simulink model "Auto_microgrid_forecasting_020322"  (R2020a)
settings: Solver=VariableStepAuto  StartTime=0.0  StopTime=10  MaxStep=1e-4  RelTol=1e-3
PreLoadFcn:
  | %run('FC_microgrid_param.m')
  | %load('gen_grid_init.mat')
InitFcn:
  | %load myisoModel_init;
  | run('FC_microgrid_param.m')
  | tic
  | run('CARTinitFcn.m')
  | %caseNo = 2;
  | 
  | %if (caseNo == 1)
  | %set_param(['Isolated_grid_paper_model_022521/SignalGen'], 'ActiveScenario', 'PStep222kW');
  | %else
  | %set_param(['Isolated_grid_paper_model_022521/SignalGen'], 'ActiveScenario', 'QStep222kVAr');
  | 
  | %end;
StopFcn:
  | toc
undefined symbols (not defined in the file or in its folder): breakpoints1, breakpoints2, cc_kp, cp_table_data, ctrl, D1, Delta, DiscIntNeverNeededParam, DT, FC_BESS, FC_PV_FirstSolar, find_system, Fnom, gcbh, libFC_BESS, libFC_PV, LowerLimit, magnitude, oversize, pll_ki, pll_kp, pq_ts, SOC_target, sps_rtmsupport, timer, Ts, ts, Ts_APC, Ts_Control, Ts_Power, UpperLimit
libraries: powerlib x151, simulink x100, powerlib_extras x100, powerlib_meascontrol x91, eePowerMeasurement x26, pi_ctrl x16, simulink_extras x12, sps_avr x7, spsDieselMotorModel x3, libFSArray x2, SignalEditorBlockLib x2, libLgBattery x1
(part 7 of 14)

== system Auto_microgrid_forecasting_020322/Stab1/AllStringInverters/Subsystem1 ==
  SmaINV : powerlib/Measurements/Three-Phase V-I Measurement  VoltageMeasurement=phase-to-ground  SetLabelV=off  LabelV=circuit_Usmainv  Vpu=off  VpuLL=off  CurrentMeasurement=yes  SetLabelI=off  LabelI=circuit_Ismainv  Ipu=off  Pbase=100e6  Vbase=500e3  OutputType=Complex  PhasorSimulation=off  PSBequivalent=0
  A : PMIOPort  Side=Left
  a : PMIOPort  Port=2  Side=Right
  B : PMIOPort  Port=3  Side=Left
  b : PMIOPort  Port=4  Side=Right
  C : PMIOPort  Port=5  Side=Left
  c : PMIOPort  Port=6  Side=Right
  tag scope: Iinv=scoped, Uinv=scoped
  wires:
  SmaINV/2 -> [Iinv]
  SmaINV/1 -> [Uinv]
  connections:
  A/RConn1 -- SmaINV/LConn1
  SmaINV/RConn3 -- c/RConn1
  SmaINV/RConn2 -- b/RConn1
  SmaINV/LConn2 -- B/RConn1
  C/RConn1 -- SmaINV/LConn3
  SmaINV/RConn1 -- a/RConn1

== system Auto_microgrid_forecasting_020322/Stab1/AllStringInverters/Subsystem2 ==
  GRI1 : powerlib/Measurements/Three-Phase V-I Measurement  VoltageMeasurement=phase-to-ground  SetLabelV=off  LabelV=Ugri  Vpu=off  VpuLL=off  CurrentMeasurement=yes  SetLabelI=off  LabelI=Igri  Ipu=off  Pbase=100e6  Vbase=500e3  OutputType=Complex  PhasorSimulation=off  PSBequivalent=0
  A : PMIOPort  Side=Left
  B : PMIOPort  Port=2  Side=Left
  a : PMIOPort  Port=3  Side=Right
  b : PMIOPort  Port=4  Side=Right
  C : PMIOPort  Port=5  Side=Left
  c : PMIOPort  Port=6  Side=Right
  tag scope: Igri=scoped, Ugri=scoped
  wires:
  GRI1/2 -> [Igri]
  GRI1/1 -> [Ugri]
  connections:
  GRI1/RConn1 -- a/RConn1
  GRI1/LConn1 -- A/RConn1
  GRI1/RConn2 -- b/RConn1
  GRI1/RConn3 -- c/RConn1
  GRI1/LConn2 -- B/RConn1
  GRI1/LConn3 -- C/RConn1

== system Auto_microgrid_forecasting_020322/Wind Turbine Type 4/APC (atomic)1/Baseline ==
  Action Port : ActionPort  ActionPortLabel=case [ 6 ]:
  Constant1 : Constant  Value=0
  Qcmd : Outport
  dP : Outport  Port=2
  dT : Outport  Port=3
  wires:
  Constant1/1 -> dP/1, dT/1, Qcmd/1

== system Auto_microgrid_forecasting_020322/Wind Turbine Type 4/APC (atomic)1/Inertial Response (to df) ==
  Freq (Hz) : Inport
  type1 : Inport  Port=2
  wg (pu) : Inport  Port=3
  f_setpoint : Inport  Port=4
  Action Port : ActionPort  ActionPortLabel=case [ 1 ]:
  Constant1 : Constant  Value=0
  Constant2 : Constant  Value=0
  Constant3 : Constant  Value=1e-3
  Display{3..4,6..7} (4 alike) : Display
  Divide1 : Product  Inputs=*/
  FBIC : Subsystem
  Gain : Gain  Gain=Fnom
  Lock2 : Subsystem
  Rate Limiter1 : RateLimiter  RisingSlewLimit=0.45  SampleTimeMode=inherited
  Relational Operator3 : RelationalOperator  OutDataTypeStr=boolean  RndMeth=Nearest
  Relational Operator4 : RelationalOperator  Operator=<=  OutDataTypeStr=boolean  RndMeth=Nearest
  Saturation : Saturate  UpperLimit=0.4  LowerLimit=0
  Saturation1 : Saturate  UpperLimit=1  LowerLimit=1e-5
  Scope : Scope  NumInputPorts=3
  Sum1 : Sum  Inputs=|-+
  Switch1 : Switch  Criteria=u2 > Threshold  Threshold=1
  TLIC : Subsystem  TreatAsAtomicUnit=on
  Type1 : Switch  Criteria=u2 > Threshold  Threshold=0.5
  When to start IR : DigitalClock  SampleTime=-1
  dead band1 : Constant  Value=0.2
  dT : Outport
  dP : Outport  Port=2
  Qcmd : Outport  Port=3
  wires:
  Constant1/1 -> dP/1, Qcmd/1
  Constant2/1 -> Switch1/3
  When to start IR/1 -> Switch1/2
  Lock2/1(O) -> Switch1/1
  Saturation/1 -> dT/1
  wg (pu)/1 -> [Wg], FBIC/1(wg (pu))
  Switch1/1 -> Display3/1, Scope/3, [In_Act]
  type1/1 -> Type1/2
  Sum1/1 -> Relational Operator3/1, Scope/2
  FBIC/1(Delta_P FBIC1) -> Type1/3
  Type1/1 -> [Delta_P], Display6/1
  Freq (Hz)/1 -> FBIC/2(Freq (Hz)1), [Freq]
  [In_Act] -> FBIC/3(Act1), TLIC/1(Act)
  TLIC/1(Delta_P TLIC) -> Type1/1
  [Delta_P] -> Relational Operator4/1
  f_setpoint/1 -> Gain/1
  dead band1/1 -> Relational Operator3/2
  Divide1/1 -> Rate Limiter1/1
  [Wg] -> Saturation1/1
  Saturation1/1 -> Divide1/2
  Constant3/1 -> Relational Operator4/2
  Relational Operator4/1 -> Display7/1, Lock2/2(R)
  [Freq] -> Sum1/1, Display4/1
  [Delta_P] -> Divide1/1, Scope/1
  Relational Operator3/1 -> Lock2/1(I)
  Rate Limiter1/1 -> Saturation/1
  Gain/1 -> Sum1/2

== system Auto_microgrid_forecasting_020322/Wind Turbine Type 4/APC (atomic)1/PFR ==
  Freq (Hz) : Inport
  f_setpoint : Inport  Port=2
  Action Port : ActionPort  ActionPortLabel=case [ 2 ]:
  Constant1 : Constant  Value=0
  Dead Zone : DeadZone  LowerValue=-db/60  UpperValue=db/60  SaturateOnIntegerOverflow=on
  Divide1 : Product  Inputs=*/
  Gain : Gain  Gain=Fnom
  P/f gain : Gain  Gain=1/k
  Saturation : Saturate  UpperLimit=0
  Sum : Sum  Inputs=|+-
  Sum1 : Sum  Inputs=|-+
  curtailment pu : Constant  Value=0.2
  dP : Outport
  dT : Outport  Port=2
  Qcmd : Outport  Port=3
  wires:
  Sum/1 -> Saturation/1
  Constant1/1 -> dT/1, Qcmd/1
  Saturation/1 -> dP/1
  P/f gain/1 -> Sum/1
  curtailment pu/1 -> Sum/2
  Dead Zone/1 -> P/f gain/1
  f_setpoint/1 -> Gain/1
  Freq (Hz)/1 -> Sum1/1
  Divide1/1 -> Dead Zone/1  "delta f pu"
  Sum1/1 -> Divide1/1
  Gain/1 -> Sum1/2, Divide1/2

== system Auto_microgrid_forecasting_020322/Wind Turbine Type 4/APC (atomic)1/PQ ==
  SFRcmd : Inport
  Qin : Inport  Port=2
  Action Port : ActionPort  ActionPortLabel=case [ 3 ]:
  Constant : Constant
  Constant1 : Constant  Value=0
  Sum : Sum  Inputs=|+-
  dP : Outport
  Qcmd : Outport  Port=2
  dT : Outport  Port=3
  wires:
  Constant1/1 -> dT/1
  Qin/1 -> Qcmd/1
  Constant/1 -> Sum/2
  Sum/1 -> dP/1
  SFRcmd/1 -> Sum/1

== system Auto_microgrid_forecasting_020322/Wind Turbine Type 4/APC (atomic)1/VR (handled by FRT) ==
  Action Port : ActionPort  ActionPortLabel=case [ 4 5 ]:
  Constant1 : Constant  Value=0
  Qcmd : Outport
  dP : Outport  Port=2
  dT : Outport  Port=3
  wires:
  Constant1/1 -> Qcmd/1, dT/1, dP/1

== system Auto_microgrid_forecasting_020322/Wind Turbine Type 4/Control/Excitation Control system ==
  Flux : Inport
  wr : Inport  Port=2
  Discrete PI Controller : Subsystem  DialogController=POWERSYS.PowerSysDialog  mask(Discrete PI Controller){Kp=Kp_field, Ki=Ki_field, Par_Limits=[1 0]*Vf_limit, Init=init(9), Ts=Ts}
      mask prompts: Kp "Proportional gain (Kp):"; Ki "Integral gain (Ki):"; Par_Limits "Output limits: [ Upper   Lower ]"; Init "Output initial value:"; Ts "Sample time:"
      mask help: This block implements a discrete PI controller.
      mask init:
      | UpperLimit=Par_Limits(1);
      | LowerLimit=Par_Limits(2);
      | power_initmask();
      mask Help: This block is part of a subset of blocks in the Extras library that does not have documentation associated with it, other than the block mask description.
      mask Display: disp('PI');
  Divide : Product  Inputs=*/
  Flux_ref : Constant
  "Flux_ref " : Constant
  Sum4 : Sum  Inputs=|+-  InputSameDT=on  SaturateOnIntegerOverflow=on  OutDataTypeStr=Inherit: Same as first input
  Switch : Switch  Threshold=1
  avoid division by 0 : Saturate  UpperLimit=inf  LowerLimit=1e-6
  Vf : Outport  VectorParamsAs1DForOutWhenUnconnected=off
  wires:
  Sum4/1 -> Discrete PI Controller/1(Error)
  Discrete PI Controller/1(Out) -> Vf/1  "Vf"
  Flux/1 -> Sum4/2  "Flux"
  wr/1 -> Switch/2, avoid division by 0/1
  Flux_ref/1 -> Switch/3
  "Flux_ref "/1 -> Divide/1
  avoid division by 0/1 -> Divide/2
  Divide/1 -> Switch/1
  Switch/1 -> Sum4/1

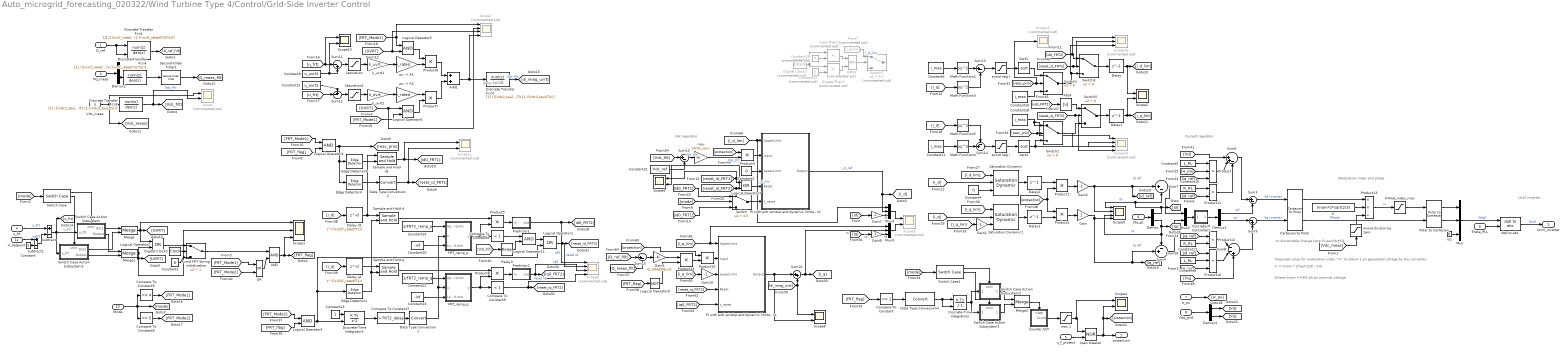
== system Auto_microgrid_forecasting_020322/Wind Turbine Type 4/Control/Grid-Side Inverter Control ==
  note: no discernable change here if use Vdc_filt
  note: di for FRT
  note: Required value for modulation index "m" to obtain 1 pu generated voltage by the converter:
  note: Modulation index and phase
  note: Where Vnom = RMS ph-ph nominal voltage
  note: Uctrl inverter
  note: Current regulator
  note: Iq ref
  note: m = Vnom * 2*sqrt(2/3) / Vdc
  note: Id ref
  note: Vdc regulator
  Q_ref : Inport
  PQ_meas : Inport  Port=2
  Vdc_meas : Inport  Port=3
  u_frt : Inport  Port=4
  u_f_protect : Inport  Port=5
  Idq_gc : Inport  Port=6
  w_pu : Inport  Port=7
  Vdq_grid : Inport  Port=8
  Theta_PLL : Inport  Port=9
  Mode : Inport  Port=10
  V_Setpoint : Inport  Port=11
  ->pu : Gain  Gain=1/Vdc_nom
  0-Mod_index_max : Saturate  UpperLimit=Mod_index_max  LowerLimit=0
  AND : Logic  IconShape=distinctive  AllPortsSameDT=off  OutDataTypeStr=boolean
  AND3 : Logic  Commented=on  IconShape=distinctive  AllPortsSameDT=off  OutDataTypeStr=boolean
  Abs4 : Abs
  Add1 : Sum
  Avoid FRT during initialization : Switch  Criteria=u2 > Threshold  Threshold=1
  Avoid division by zero : Saturate  UpperLimit=1e6  LowerLimit=1e-6
  Cartesian to Polar : simulink_extras/Transformations/Cartesian to Polar
  Compare To Constant : simulink/Logic and Bit Operations/Compare To Constant  relop===  const=1  OutDataTypeStr=boolean
  Compare To Constant5 : simulink/Logic and Bit Operations/Compare To Constant  relop===  const=4  OutDataTypeStr=boolean
  Compare To Constant6 : simulink/Logic and Bit Operations/Compare To Constant  relop===  const=5  OutDataTypeStr=boolean
  Compare To Constant7 : simulink/Logic and Bit Operations/Compare To Constant  relop=>  const=FRT2_delay  OutDataTypeStr=boolean
  Compare To Constant8 : simulink/Logic and Bit Operations/Compare To Constant  relop=<  const=1  OutDataTypeStr=boolean
  Compare To Constant9 : simulink/Logic and Bit Operations/Compare To Constant  relop=<  const=1  OutDataTypeStr=boolean
  Constant : Constant
  Constant10 : Constant  Value=R_RL
  Constant{6,11,16,18} (4 alike) : Constant  Value=i_max  SampleTime=Ts
  Constant12 : Constant  Value=u_ovrt1  SampleTime=Ts
  Constant13 : Constant
  Constant17 : Constant  Value=R_RL
  Constant19 : Constant  Value=1/FRT2_ramp_p  SampleTime=Ts
  Constant2 : Constant  Value=0  SampleTime=Ts
  Constant20 : Constant  Value=-inf  SampleTime=Ts
  Constant21 : Constant  Value=Vdc_ref  SampleTime=Ts
  Constant22 : Constant  Value=1/FRT2_ramp_q  SampleTime=Ts
  Constant23 : Constant  Value=-inf  SampleTime=Ts
  Constant27 : Constant  Commented=on  Value=2
  Constant28 : Constant  Commented=on  Value=7
  Constant3 : Constant  Value=0
  Constant4 : Constant  Value=0  SampleTime=Ts
  Constant5 : Constant  Value=L_RL
  Constant8 : Constant  Value=L_RL
  Constant9 : Constant  Value=u_uvrt1  SampleTime=Ts
  Counter AST : Subsystem
  Data Type Conversion1 : DataTypeConversion
  Data Type Conversion2 : DataTypeConversion
  Data Type Conversion4 : DataTypeConversion
  Delay{,1..3} (4 alike) : Delay  DelayLength=1  InitialCondition=0  SampleTime=Ts
  Delay d1 : Delay  DelayLength=fix(2/(f_rated*Ts))  InitialCondition=1  SampleTime=Ts
  Delay q1 : Delay  DelayLength=fix(2/(f_rated*Ts))  InitialCondition=1  SampleTime=Ts
  Demux{,2..4} (4 alike) : Demux  Outputs=2
      Demux settings: DisplayOption=none
      Demux3 settings: DisplayOption=none
      Demux4 settings: DisplayOption=none
  Digital Clock2 : DigitalClock  SampleTime=Ts
  Digital Clock3 : DigitalClock  Commented=on  SampleTime=-1
  Discrete PI Controller1 : Subsystem  DialogController=POWERSYS.PowerSysDialog  mask(Discrete PI Controller){Kp=Kp_grid_side_cur_reg, Ki=Ki_grid_side_cur_reg, Par_Limits=[1 -1]*Current_reg_output_limit, Init=0, Ts=Ts}
      mask prompts: Kp "Proportional gain (Kp):"; Ki "Integral gain (Ki):"; Par_Limits "Output limits: [ Upper   Lower ]"; Init "Output initial value:"; Ts "Sample time:"
      mask help: This block implements a discrete PI controller.
      mask init:
      | UpperLimit=Par_Limits(1);
      | LowerLimit=Par_Limits(2);
      | power_initmask();
      mask Help: This block is part of a subset of blocks in the Extras library that does not have documentation associated with it, other than the block mask description.
      mask Display: disp('PI');
  Discrete Transfer Fcn1 : DiscreteTransferFcn  Denominator=[(inv(f_rated)*2)/Ts (1-((inv(f_rated)*2)/Ts))]  InitialStatesSource=Input port  SampleTime=Ts
      settings: InputPortMap=u0,p5
  Discrete Transfer Fcn2 : DiscreteTransferFcn  Denominator=[(Vdc2_tau)/Ts (1-((Vdc2_tau)/Ts))]  InitialStates=Vdc2_filt_init  SampleTime=Ts
  Discrete Transfer Fcn3 : DiscreteTransferFcn  Denominator=[(Vdc2_tau)/Ts (1-((Vdc2_tau)/Ts))]  SampleTime=Ts
  Discrete Transfer Fcn4 : DiscreteTransferFcn  Denominator=[(inv(f_rated)*2)/Ts (1-((inv(f_rated)*2)/Ts))]  InitialStates=U_rated^2/(-inv(2*pi*f_rated*Cshunt_filter))  SampleTime=Ts
  Discrete-Time Integrator2 : DiscreteIntegrator  ExternalReset=falling  SampleTime=Ts  ICPrevOutput=DiscIntNeverNeededParam  ICPrevScaledInput=DiscIntNeverNeededParam
  Discrete-Time Integrator3 : DiscreteIntegrator  ExternalReset=level  SampleTime=Ts  LimitOutput=on  UpperSaturationLimit=1  LowerSaturationLimit=0  ICPrevOutput=DiscIntNeverNeededParam  ICPrevScaledInput=DiscIntNeverNeededParam
  Edge Detector1 : powerlib_meascontrol/Logic/Edge Detector  model=Rising  ic=0  Ts=Ts
      settings: SourceProductBaseCode=PS
  Edge Detector3 : powerlib_meascontrol/Logic/Edge Detector  model=Rising  ic=0  Ts=Ts
      settings: SourceProductBaseCode=PS
  Edge Detector4 : powerlib_meascontrol/Logic/Edge Detector  model=Falling  ic=0  Ts=Ts
      settings: SourceProductBaseCode=PS
  FRT_ramp_p : Subsystem
  FRT_ramp_q : Subsystem
  From7 : From  Commented=on  GotoTag=i_d_lim
  Gain : Gain
  Gain{1..2,7,10} (4 alike) : Gain  Gain=-1
  Gain5 : Gain  Gain=Q_rated/Nb_wt
  Gain9 : Gain
  GreaterThan2 : RelationalOperator  Commented=on  Operator=>  OutDataTypeStr=boolean  RndMeth=Simplest
  K : Constant  Value=Vnom*2*sqrt(2/3)
  Less Than2 : RelationalOperator  Commented=on  Operator=<  OutDataTypeStr=boolean  RndMeth=Simplest
  Logical Operator1 : Logic  Operator=OR  AllPortsSameDT=off  OutDataTypeStr=boolean
  Logical Operator{3..6,11} (5 alike) : Logic  AllPortsSameDT=off  OutDataTypeStr=boolean
  Logical Operator2 : Logic  Operator=OR  AllPortsSameDT=off  OutDataTypeStr=boolean
  Logical Operator7 : Logic  Operator=OR  AllPortsSameDT=off  OutDataTypeStr=boolean
  Logical Operator9 : Logic  Operator=NOT  AllPortsSameDT=off  OutDataTypeStr=boolean
  Math Function{2..5} (4 alike) : Math  Operator=magnitude^2  SignedPower=on  SaturateOnIntegerOverflow=on
  Merge : Merge
  Merge1 : Merge
  Merge2 : Merge
  Mux : Mux  Inputs=3
  Mux2 : Mux  Inputs=2
  Mux3 : Mux  Inputs=3
  Mux4 : Mux  Inputs=3
  OR : Logic  Operator=OR  IconShape=distinctive  AllPortsSameDT=off  OutDataTypeStr=boolean
  PI with anti-windup and dynamic limits - Id : Subsystem  mask(Discrete PI Controller with anti-windup and dynamic limiters){Kp=Kp_dc, Ki=Ki_dc, Init=Vdc_nom, Ts=Ts}
      mask prompts: Kp "Proportional gain (Kp):"; Ki "Integral gain (Ki):"; Init "State initial value:"; Ts "Sample time:"
      mask Display:
      | disp('PI-\nAST');
      | port_label('input',1,'Max');
      | port_label('input',2,'In');
      | port_label('input',3,'Min');
      | port_label('input',4,'Reset');
      | port_label('input',5,'x_reset');
      | port_label('output',1,'Out');
  PI with anti-windup and dynamic limits - Iq : Subsystem  mask(Discrete PI Controller with anti-windup and dynamic limiters){Kp=Q_Kp/1000, Ki=Q_Ki/1000, Init=0, Ts=Ts}
      mask prompts: Kp "Proportional gain (Kp):"; Ki "Integral gain (Ki):"; Init "State initial value:"; Ts "Sample time:"
      mask Display:
      | disp('PI-\nAST');
      | port_label('input',1,'Max');
      | port_label('input',2,'In');
      | port_label('input',3,'Min');
      | port_label('input',4,'Reset');
      | port_label('input',5,'x_reset');
      | port_label('output',1,'Out');
  Polar to Cartesian : simulink_extras/Transformations/Polar to Cartesian
      settings: SourceProductBaseCode=SL
  Predictor1 : Subsystem  mask{Init_value=0, Ts=Ts}
      mask prompts: Init_value "Initial value:"; Ts "Sample time (Ts):"
  Predictor2 : Subsystem  mask{Init_value=0, Ts=Ts}
      mask prompts: Init_value "Initial value:"; Ts "Sample time (Ts):"
  Product : Product  Inputs=3  InputSameDT=on  SaturateOnIntegerOverflow=on  OutDataTypeStr=Inherit: Same as first input
  Product{1..2,4..8,14..15} (9 alike) : Product
  Product10 : Product  Inputs=3  InputSameDT=on  SaturateOnIntegerOverflow=on  OutDataTypeStr=Inherit: Same as first input
  Product11 : Product  InputSameDT=on  SaturateOnIntegerOverflow=on  OutDataTypeStr=Inherit: Same as first input
  Product12 : Product  InputSameDT=on  SaturateOnIntegerOverflow=on  OutDataTypeStr=Inherit: Same as first input
  Product13 : Product  Inputs=**/  InputSameDT=on  SaturateOnIntegerOverflow=on  OutDataTypeStr=Inherit: Same as first input
  Relay3 : Relay  OnSwitchValue=1.02*Vdc_ref  OffSwitchValue=1.015*Vdc_ref  OutDataTypeStr=Inherit: Inherit via back propagation
  Sample and Hold d : powerlib_meascontrol/Additional Components/Sample and Hold  ic=0  Ts=Ts
      settings: SourceProductBaseCode=PS
  Sample and Hold d1 : powerlib_meascontrol/Additional Components/Sample and Hold  ic=0  Ts=Ts
      settings: SourceProductBaseCode=PS
  Sample and Hold q : powerlib_meascontrol/Additional Components/Sample and Hold  ic=0  Ts=Ts
      settings: SourceProductBaseCode=PS
  Saturation : Saturate  UpperLimit=0.08  LowerLimit=0
  Saturation Dynamic : simulink/Discontinuities/Saturation Dynamic  OutMin=[]  OutMax=[]  OutDataTypeStr=Inherit: Same as second input  OutDataType=fixdt(1, 16)  OutScaling=2^-10  DoSatur=off
  Saturation Dynamic1 : simulink/Discontinuities/Saturation Dynamic  OutMin=[]  OutMax=[]  OutDataTypeStr=Inherit: Same as second input  OutDataType=fixdt(1, 16)  OutScaling=2^-10  DoSatur=off
  Saturation1 : Saturate  UpperLimit=0  LowerLimit=-0.08
  Scope : Scope  Commented=on  NumInputPorts=2
  Scope1 : Scope  NumInputPorts=3
  Scope10 : Scope  Commented=on  NumInputPorts=4
  Scope11 : Scope  Commented=on  NumInputPorts=2
  Scope{2,4,6,9,13} (5 alike) : Scope  NumInputPorts=2
  Scope15 : Scope  Commented=on
  Scope16 : Scope  Commented=on  NumInputPorts=3
  Scope3 : Scope  Commented=on  NumInputPorts=2
  Scope5 : Scope  NumInputPorts=4
  Scope7 : Scope  Commented=on  NumInputPorts=4
  Scope8 : Scope  Commented=on  NumInputPorts=4
  Second-Order Filter1 : powerlib_meascontrol/Filters/Second-Order Filter  FilterType=Lowpass  Fo=Freq_filter  Zeta=Zeta_filter  Ts=Ts  Initialize=off  Vac_Init="[0,  0,  60]"  Vdc_Init=0  PlotResponse=off  FreqRange=[0, 500, 1]
      settings: SourceProductBaseCode=MT,PS
  Sqrt1 : Sqrt  SaturateOnIntegerOverflow=on
  Sqrt2 : Sqrt  SaturateOnIntegerOverflow=on
  Subtract : Sum  Inputs=+-
  Subtract1 : Sum  Inputs=+-
  Sum10 : Sum  Inputs=|+-
  Sum11 : Sum  Inputs=|-+
  Sum12 : Sum  Inputs=+-|
  Sum13 : Sum  Inputs=|+-
  Sum14 : Sum  Inputs=-+|
  Sum15 : Sum  Inputs=|+-
  Sum16 : Sum  Inputs=|++
  Sum3 : Sum  Inputs=|+-  InputSameDT=on  SaturateOnIntegerOverflow=on  OutDataTypeStr=Inherit: Same as first input
  Sum4 : Sum  Inputs=-+|  InputSameDT=on  SaturateOnIntegerOverflow=on  OutDataTypeStr=Inherit: Same as first input
  Sum6 : Sum  Inputs=||++-  InputSameDT=on  SaturateOnIntegerOverflow=on  OutDataTypeStr=Inherit: Same as first input
  Sum7 : Sum  Inputs=|+-  InputSameDT=on  SaturateOnIntegerOverflow=on  OutDataTypeStr=Inherit: Same as first input
  Sum8 : Sum  Inputs=|--+  InputSameDT=on  SaturateOnIntegerOverflow=on  OutDataTypeStr=Inherit: Same as first input
  Sum9 : Sum  Inputs=|-+  InputSameDT=on  SaturateOnIntegerOverflow=on  OutDataTypeStr=Inherit: Same as first input
  Switch : Switch  Criteria=u2 > Threshold  Threshold=4.5
  Switch Case : SwitchCase  CaseConditions={4, 5}
  Switch Case Action Subsystem : Subsystem  TreatAsAtomicUnit=on
  Switch Case Action Subsystem1 : Subsystem  TreatAsAtomicUnit=on
  Switch Case Action Subsystem2 : Subsystem  TreatAsAtomicUnit=on
  Switch Case Action Subsystem3 : Subsystem  TreatAsAtomicUnit=on
  Switch Case1 : SwitchCase  CaseConditions={4, 5}
  Switch{1..3,5} (4 alike) : Switch  Criteria=u2 > Threshold
  Switch7 : Switch  Commented=on  Criteria=u2 > Threshold  Threshold=0.5
  V0 : Constant  Value=0
  avoid neg i : Saturate  UpperLimit=i_max^2  LowerLimit=0
  avoid neg r : Saturate  UpperLimit=i_max^2  LowerLimit=0
  dq0 to abc : powerlib_meascontrol/Transformations/dq0 to abc  Alignment=90 degrees behind phase A axis
      settings: SourceProductBaseCode=MT,PS
  k_uvrt1 : Gain  Gain=k_uvrt
  k_uvrt2 : Gain  Gain=k_ovrt
  max 1 : Saturate  UpperLimit=1  LowerLimit=0
  open breaker : Logic  Operator=NOR  AllPortsSameDT=off  OutDataTypeStr=boolean
  "pu -> A1" : Gain  Gain=i_rated
  "pu -> A2" : Gain  Gain=i_rated
  protection : Outport
  Uctrl_inverter : Outport  Port=2  VectorParamsAs1DForOutWhenUnconnected=off
  wires:
  Logical Operator5/1 -> Product6/1
  [UVRT] -> Scope7/3, Logical Operator5/2
  [FRT_Mode1] -> Scope7/1, Logical Operator5/1
  Q_ref/1 -> Discrete Transfer Fcn1/1, Discrete Transfer Fcn1/2
  Discrete Transfer Fcn1/1 -> [Q_ref_filt]
  Product7/1 -> Add1/2
  "pu -> A2"/1 -> Product7/1
  Logical Operator6/1 -> Product7/2
  [FRT_Mode1] -> Logical Operator6/2
  [OVRT] -> Scope7/2, Logical Operator6/1
  Sum12/1 -> Saturation1/1
  k_uvrt2/1 -> "pu -> A2"/1
  Compare To Constant6/1 -> [FRT_Mode2]
  Compare To Constant5/1 -> [FRT_Mode1]
  [u_frt] -> Sum12/2
  Constant12/1 -> Sum12/1
  Add1/1 -> Scope7/4, Discrete Transfer Fcn3/1
  Product6/1 -> Add1/1
  "pu -> A1"/1 -> Product6/2
  Sum11/1 -> Saturation/1
  k_uvrt1/1 -> "pu -> A1"/1
  [u_frt] -> Scope13/1, Sum11/1
  Constant9/1 -> Scope13/2, Sum11/2
  Vdc_meas/1 -> Discrete Transfer Fcn2/1, Scope/1, [Vdc_meas]
  Discrete Transfer Fcn2/1 -> Scope/2, [Vdc_filt]  "Vdc_filt"
  Subtract/1 -> [u_frt], Switch Case Action Subsystem1/1(u_frt), Switch Case Action Subsystem/1(u_frt)  "u_Frt"
  Avoid FRT during initialization/1 -> AND/1
  avoid neg r/1 -> Sqrt1/1
  avoid neg i/1 -> Sqrt2/1
  [i_q] -> Math Function3/1
  [reac_prio] -> Scope10/3, Switch2/2
  Sqrt2/1 -> Scope10/2, Switch2/3
  Constant18/1 -> Scope10/1, Switch2/1
  [reac_prio] -> Scope15/1, Switch1/2
  Constant16/1 -> Switch1/3
  Sqrt1/1 -> Switch1/1
  [i_d] -> Math Function5/1
  Sum14/1 -> avoid neg i/1
  Constant11/1 -> Math Function4/1
  Sum13/1 -> avoid neg r/1
  Math Function3/1 -> Sum13/2
  Math Function2/1 -> Sum13/1
  Constant6/1 -> Math Function2/1
  Math Function4/1 -> Sum14/2
  Math Function5/1 -> Sum14/1
  Switch1/1 -> Switch3/3, Scope16/3
  Switch3/1 -> Delay/1
  [id0_FRT2] -> Scope16/1, Switch3/1
  [reset_id_FRT2] -> Scope16/2, Switch3/2
  Switch2/1 -> Switch5/3
  [iq0_FRT2] -> Abs4/1
  [reset_iq_FRT2] -> Scope10/4, Switch5/2
  Switch5/1 -> Delay1/1
  Delay/1 -> Scope2/1, [i_d_lim]
  Delay1/1 -> Scope2/2, [i_q_lim]
  Constant2/1 -> PI with anti-windup and dynamic limits - Id/3(LowerLimit)
  [i_q_lim] -> Gain1/1
  [i_q_lim] -> Saturation Dynamic1/1
  Gain1/1 -> Saturation Dynamic1/3
  [i_d_lim] -> Saturation Dynamic/1
  Saturation Dynamic1/1 -> Delay3/1
  Saturation Dynamic/1 -> Delay2/1
  Constant4/1 -> Saturation Dynamic/3
  PQ_meas/1 -> Demux2/1
  [i_d_lim] -> Mux4/1, PI with anti-windup and dynamic limits - Id/1(UpperLimit)  "i_d_lim"
  Demux2/2 -> Discrete Transfer Fcn4/1
  Abs4/1 -> Switch5/1
  [FRT_flag] -> Compare To Constant/1
  Discrete-Time Integrator2/1 -> Switch Case Action Subsystem2/1(u_frt), Switch Case Action Subsystem3/1(u_frt)
  Data Type Conversion4/1 -> Discrete-Time Integrator2/2, Discrete-Time Integrator2/1
  Merge2/1 -> Counter AST/Trigger
  Counter AST/1(Count) -> max 1/1
  Compare To Constant/1 -> Data Type Conversion4/1
  max 1/1 -> Scope4/1, open breaker/1
  u_f_protect/1 -> open breaker/2
  open breaker/1 -> protection/1, Scope4/2, [protection]
  [FRT_Mode2] -> Logical Operator4/1
  [FRT_flag] -> Logical Operator4/2
  [i_d] -> Delay d1/1
  [i_q] -> Delay q1/1
  Delay d1/1 -> Sample and Hold d1/1, Sample and Hold d/1
  Delay q1/1 -> Sample and Hold q/1
  Edge Detector1/1 -> Sample and Hold d/2, Sample and Hold q/2
  Constant13/1 -> Discrete-Time Integrator3/1
  Discrete-Time Integrator3/1 -> Compare To Constant7/1
  Compare To Constant7/1 -> Data Type Conversion1/1
  Product5/1 -> Predictor1/1(in)
  Product8/1 -> Predictor2/1(in)
  Sample and Hold q/1 -> Product8/1
  Predictor2/1(out) -> Scope8/3, [iq0_FRT2]  "iq0"
  FRT_ramp_q/1(y) -> Compare To Constant9/1, Product8/2
  Compare To Constant9/1 -> Scope8/4, [reset_iq_FRT2]  "reset iq"
  FRT_ramp_p/1(y) -> Compare To Constant8/1, Product5/2
  [Vdc_filt] -> Relay3/1
  Compare To Constant8/1 -> Logical Operator11/1
  Logical Operator11/1 -> Logical Operator1/1
  Logical Operator4/1 -> Discrete-Time Integrator3/2, Logical Operator1/2, Edge Detector1/1
  Logical Operator1/1 -> Scope8/2, [reset_id_FRT2]  "reset id"
  Data Type Conversion1/1 -> FRT_ramp_q/2(u), FRT_ramp_p/2(u)
  Relay3/1 -> Logical Operator11/2
  Constant19/1 -> FRT_ramp_p/1(UpperLimit)
  Constant20/1 -> FRT_ramp_p/3(LowerLimit)
  Constant22/1 -> FRT_ramp_q/1(UpperLimit)
  Constant23/1 -> FRT_ramp_q/3(LowerLimit)
  Switch/1 -> PI with anti-windup and dynamic limits - Id/5(x_reset)
  [FRT_Mode1] -> Logical Operator3/1
  [FRT_flag] -> Logical Operator3/2
  Logical Operator3/1 -> Edge Detector4/1, Edge Detector3/1, [reac_prio]
  Edge Detector3/1 -> Sample and Hold d1/2
  Sample and Hold d1/1 -> [id0_FRT1], Scope11/1
  Edge Detector4/1 -> Data Type Conversion2/1
  Data Type Conversion2/1 -> Scope11/2, [reset_id_FRT1]
  [reset_id_FRT1] -> Logical Operator7/1, Scope9/1
  [reset_id_FRT2] -> Scope9/2, Logical Operator7/2
  Logical Operator7/1 -> PI with anti-windup and dynamic limits - Id/4(Reset)
  [mode] -> Switch/2
  [id0_FRT1] -> Switch/3
  [id0_FRT2] -> Switch/1
  Predictor1/1(out) -> Scope8/1, [id0_FRT2]  "id0"
  Delay2/1 -> Product1/1
  Delay3/1 -> Product2/2
  [protection] -> Product2/1, Product1/2
  Product2/1 -> Gain/1
  Product4/1 -> PI with anti-windup and dynamic limits - Id/2(Input)
  [protection] -> Product4/1
  [i_d] -> Saturation Dynamic/2
  [i_q] -> Saturation Dynamic1/2
  Sample and Hold d/1 -> Product5/1
  Logical Operator2/1 -> Avoid FRT during initialization/1
  Constant3/1 -> Avoid FRT during initialization/3
  Digital Clock2/1 -> Avoid FRT during initialization/2
  [Vdc_meas] -> Avoid division by zero/1
  Cartesian to Polar/1 -> Product13/1
  Product13/1 -> 0-Mod_index_max/1  "m"
  Demux4/1 -> [Vd]
  w_pu/1 -> [w_pu]
  [iq_ref] -> Product/3
  Sum7/1 -> Mux2/1
  [w_pu] -> Product/2
  Product11/1 -> Sum6/3
  Avoid division by zero/1 -> Product13/3
  Product12/1 -> Sum8/1
  Demux3/2 -> Sum9/1  "vq'"
  Constant10/1 -> Product11/1
  Discrete PI Controller1/1(Out) -> Demux3/1
  Mux2/1 -> Discrete PI Controller1/1(Error)
  Product/1 -> Sum6/2
  Product1/1 -> Gain2/1
  Vdq_grid/1 -> Demux4/1
  Gain/1 -> Sum4/2, [iq_ref], Scope5/4
  Demux3/1 -> Sum3/2  "vd'"
  Constant8/1 -> Product10/2
  Product10/1 -> Sum8/2
  [Vd] -> Sum6/1
  Constant17/1 -> Product12/2
  [w_pu] -> Product10/3
  Sum8/1 -> Sum9/2
  Demux/1 -> Sum7/2, Scope5/1, [id]  "id"
  [id_ref] -> Product10/1
  dq0 to abc/1 -> Uctrl_inverter/1  "Uctrl"
  Polar to Cartesian/2 -> Mux/2
  Sum6/1 -> Sum3/1
  K/1 -> Product13/2
  Mux/1 -> dq0 to abc/1  "Vdq0"
  [Vq] -> Sum8/3
  Sum3/1 -> Cartesian to Polar/1  "Vd inverter"
  [iq_ref] -> Product12/1
  Cartesian to Polar/2 -> Polar to Cartesian/2  "Phase"
  0-Mod_index_max/1 -> Polar to Cartesian/1
  Sum9/1 -> Cartesian to Polar/2  "Vq inverter"
  [id_ref] -> Product11/2
  Constant5/1 -> Product/1
  Polar to Cartesian/1 -> Mux/1
  Sum4/1 -> Mux2/2
  Demux4/2 -> [Vq]
  V0/1 -> Mux/3
  Theta_PLL/1 -> dq0 to abc/2
  Idq_gc/1 -> Demux/1
  PI with anti-windup and dynamic limits - Id/1(Output) -> [i_d], Mux4/2  "i_d_ref"
  Gain2/1 -> Scope5/2, Sum7/1, [id_ref]
  ->pu/1 -> Product4/2  "Vdc_filt"
  Constant21/1 -> Sum10/2
  [Vdc_filt] -> Sum10/1
  Mux4/1 -> Scope3/1
  Mux3/1 -> Scope3/2
  Demux/2 -> Scope5/3, Sum4/1, [iq]  "iq"
  [id] -> Gain7/1
  Gain9/1 -> Mux3/3  "iq"
  Gain7/1 -> Mux4/3  "id"
  [iq] -> Gain9/1  "iq"
  [iq0_FRT2] -> PI with anti-windup and dynamic limits - Iq/5(x_reset)
  [FRT_flag] -> Logical Operator9/1
  [i_q_lim] -> Mux3/1, PI with anti-windup and dynamic limits - Iq/1(UpperLimit)
  PI with anti-windup and dynamic limits - Iq/1(Output) -> Scope6/2, Sum16/1
  Product14/1 -> Product15/2
  [Q_ref_filt] -> Sum15/1
  [reset_iq_FRT2] -> PI with anti-windup and dynamic limits - Iq/4(Reset)
  Logical Operator9/1 -> Product14/2
  Sum15/1 -> Gain5/1
  Sum16/1 -> Mux3/2, [i_q]  "iq"
  [Q_meas_filt] -> Sum15/2
  [i_q_lim] -> Gain10/1
  [di_imag_uvrt] -> Scope6/1, Sum16/2
  Product15/1 -> PI with anti-windup and dynamic limits - Iq/2(Input)
  [protection] -> Product15/1
  Gain10/1 -> PI with anti-windup and dynamic limits - Iq/3(LowerLimit)
  Saturation/1 -> k_uvrt1/1
  Saturation1/1 -> k_uvrt2/1
  Discrete Transfer Fcn3/1 -> [di_imag_uvrt]  "Vdc_filt"
  Sum10/1 -> ->pu/1  "Vdc_filt"
  Gain5/1 -> Product14/1
  Discrete Transfer Fcn4/1 -> Second-Order Filter1/1
  Second-Order Filter1/1 -> [Q_meas_filt]
  AND/1 -> Scope1/3, [FRT_flag]
  Digital Clock3/1 -> Less Than2/1, GreaterThan2/1
  Constant28/1 -> Less Than2/2
  Constant27/1 -> GreaterThan2/2
  From7/1 -> Switch7/1  "i_d_lim"
  AND3/1 -> Switch7/2
  GreaterThan2/1 -> AND3/2
  Less Than2/1 -> AND3/1
  [mode] -> Switch Case/1
  Switch Case/1 -> Switch Case Action Subsystem/Action
  Switch Case/2 -> Switch Case Action Subsystem1/Action
  Merge/1 -> Scope1/1, Logical Operator2/1, [OVRT]
  Switch Case Action Subsystem/1(Out1) -> Merge/1
  Switch Case Action Subsystem1/1(Out1) -> Merge/2
  Switch Case Action Subsystem/2(Output) -> Merge1/1
  Switch Case Action Subsystem1/2(Output) -> Merge1/2
  Merge1/1 -> Scope1/2, [UVRT], Logical Operator2/2
  Switch Case1/2 -> Switch Case Action Subsystem3/Action
  Switch Case1/1 -> Switch Case Action Subsystem2/Action
  [mode] -> Switch Case1/1
  Switch Case Action Subsystem2/1(Out1) -> Merge2/1
  Switch Case Action Subsystem3/1(Out1) -> Merge2/2
  u_frt/1 -> Subtract/1  "u_Frt"
  V_Setpoint/1 -> Subtract1/1
  Subtract1/1 -> Subtract/2  "u_Frt"
  Constant/1 -> Subtract1/2
  OR/1 -> AND/2
  Mode/1 -> [mode], Compare To Constant6/1, Compare To Constant5/1
  [FRT_Mode1] -> OR/1
  [FRT_Mode2] -> OR/2

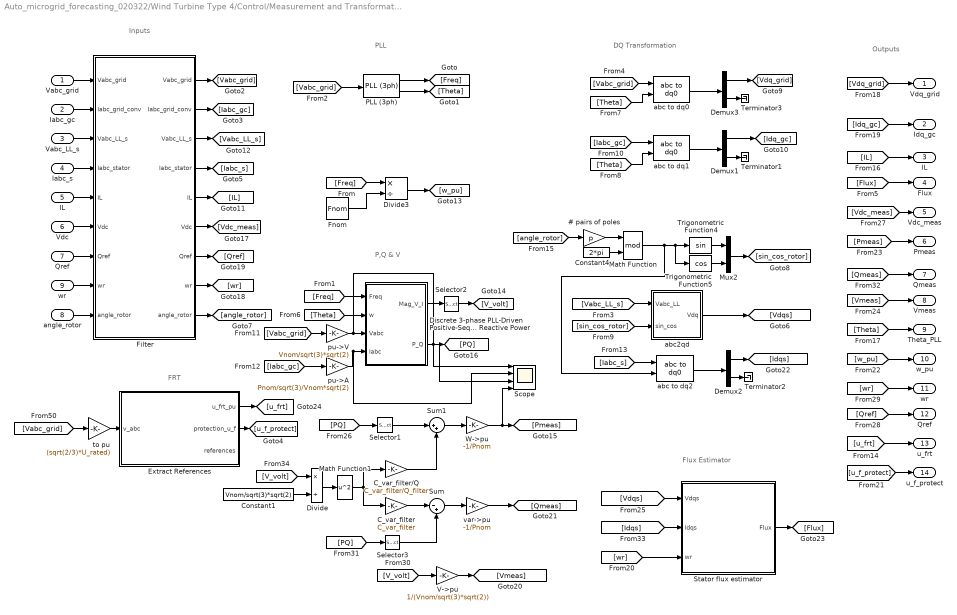
== system Auto_microgrid_forecasting_020322/Wind Turbine Type 4/Control/Measurement and Transformation ==
  note: Flux Estimator
  note: Outputs
  note: PLL
  note: DQ Transformation
  note: P,Q & V
  note: Inputs
  note: FRT
  Vabc_grid : Inport
  Iabc_gc : Inport  Port=2
  Vabc_LL_s : Inport  Port=3
  Iabc_s : Inport  Port=4
  IL : Inport  Port=5
  Vdc : Inport  Port=6
  Qref : Inport  Port=7
  angle_rotor : Inport  Port=8
  wr : Inport  Port=9
  # pairs of poles : Gain  Gain=p  SaturateOnIntegerOverflow=on  OutDataTypeStr=Inherit: Same as input  ParamDataTypeStr=Inherit: Same as input
  C_var_filter : Gain  Gain=C_var_filter  SaturateOnIntegerOverflow=on  OutDataTypeStr=Inherit: Same as input  ParamDataTypeStr=Inherit: Same as input
  C_var_filter/Q : Gain  Gain=C_var_filter/Q_filter  SaturateOnIntegerOverflow=on  OutDataTypeStr=Inherit: Same as input  ParamDataTypeStr=Inherit: Same as input
  Constant1 : Constant  Value=Vnom/sqrt(3)*sqrt(2)
  Constant4 : Constant  Value=2*pi
  Demux1 : Demux  Outputs=[2 1]
      settings: DisplayOption=none
  Demux2 : Demux  Outputs=[2 1]
      settings: DisplayOption=none
  Demux3 : Demux  Outputs=[2 1]
      settings: DisplayOption=none
  Discrete 3-phase PLL-Driven Positive-Sequence Active & Reactive Power : Subsystem  mask(Discrete 3-phase PLL-Driven Positive-Sequence Active & Reactive Power){Finit=Fnom, Fmin=Fnom*45/60, Par_Vinit=[Vnom/sqrt(3)*sqrt(2) 30], Par_Iinit=[Pnom/sqrt(3)/Vnom*sqrt(2) -10], Ts=Ts}
      mask prompts: Finit "Initial frequency (Hz):"; Fmin "Minimum frequency (Hz):"; Par_Vinit "Voltage initial input: [ Mag  Phase(Degrees) ]"; Par_Iinit "Current initial input: [ Mag  Phase(Degrees) ]"; Ts "Sample time:"
      mask help:
      | This discrete block measures the 3-phase active power P and reactive power Q  associated with a periodic set of 3-phase voltages and currents which may contain harmonics. P and Q are calculated by evaluating the fundamental values (positive-sequence) of the input voltages and currents with a running window over one cycle of the specified frequency (port Freq).
      |  Input port "Sin_Cos" (a two-dimension signal) provides the reference frame required for the computation.
      |
      | input 1: must give the frequency of the fundamental (Hz)
      | Input 2: must contain a  [sin(wt)  cos(wt)] two dimension signal , where w is the rotation speed (rad/s) of the reference frame used for the computation..
      | input 3: Vectorized 3-phase  instantaneous voltage (Vabc)
      | input 4: Vectorized 3-phase instantaneous current (Iabc)
      |
      | Output 1: Vector [Mag_V Mag_I] of the fundamental values (Magnitude) of the voltage & current (peak values of the positive-sequence)
      | Output 2: 3-phase PQ measurement vector [P(W) Q (var)] evaluated at the specified frequency. Current flowing into an RL circuit will produce  positive active and reactive powers.
      |
      | For the first cycle of simulation, the outputs are held constant using the values specified by the parameters "Initial input".
      | he value of the parameter "Minimum frequency" is used to determine the buffer size of the "Variable Transport Delay" block found inside this subsystem.
      mask init:
      | power_initmask();
      settings: OpenFcn=power_openblockproxy();
  Divide : Product  Inputs=*/
  Divide3 : Product  Inputs=*/
  Extract References : Subsystem
  Filter : Subsystem  mask{Freq=Freq_filter, Zeta=Zeta_filter, Ts=Ts}
      mask prompts: Freq "Cut-off frequency (Hz):"; Zeta "Damping factor Zeta:"; Ts "Sample time"
  Fnom : Constant  Value=Fnom
  Math Function : Math  Operator=mod  SignedPower=on  SaturateOnIntegerOverflow=on
  Math Function1 : Math  Operator=square  SignedPower=on  SaturateOnIntegerOverflow=on
  Mux2 : Mux  Inputs=2
  PLL (3ph) : powerlib_meascontrol/PLL/PLL (3ph)  Fmin=0.75*Fnom  Par_Init=[-45 Fnom]  ParK=[60 1400 1]  TcD=1e-4  MaxRateChangeFreq=12  FilterCutOffFreq=25  Ts=Ts  AGC=on
      settings: SourceProductBaseCode=MT,PS
  Scope : Scope  NumInputPorts=4
  Selector1 : Selector  InputPortWidth=2  IndexOptions=Index vector (dialog)  Indices=1  OutputSizes=1
  Selector2 : Selector  InputPortWidth=2  IndexOptions=Index vector (dialog)  Indices=1  OutputSizes=1
  Selector3 : Selector  InputPortWidth=2  IndexOptions=Index vector (dialog)  Indices=2  OutputSizes=1
  Stator flux estimator : Subsystem
  Sum : Sum  Inputs=|-+
  Sum1 : Sum  Inputs=|++
  Terminator1 : Terminator
  Terminator2 : Terminator
  Terminator3 : Terminator
  Trigonometric Function4 : Trigonometry
  Trigonometric Function5 : Trigonometry  Operator=cos
  V->pu : Gain  Gain=1/(Vnom/sqrt(3)*sqrt(2))  SaturateOnIntegerOverflow=on  OutDataTypeStr=Inherit: Same as input  ParamDataTypeStr=Inherit: Same as input
  W->pu : Gain  Gain=-1/Pnom  SaturateOnIntegerOverflow=on  OutDataTypeStr=Inherit: Same as input  ParamDataTypeStr=Inherit: Same as input
  abc to dq0 : powerlib_meascontrol/Transformations/abc to dq0  Alignment=90 degrees behind phase A axis
      settings: SourceProductBaseCode=MT,PS
  abc to dq1 : powerlib_meascontrol/Transformations/abc to dq0  Alignment=90 degrees behind phase A axis
      settings: SourceProductBaseCode=MT,PS
  abc to dq2 : powerlib_meascontrol/Transformations/abc to dq0  Alignment=90 degrees behind phase A axis
      settings: SourceProductBaseCode=MT,PS
  abc2qd : Subsystem
  pu->A : Gain  Gain=Pnom/sqrt(3)/Vnom*sqrt(2)  SaturateOnIntegerOverflow=on  OutDataTypeStr=Inherit: Same as input  ParamDataTypeStr=Inherit: Same as input
  pu->V : Gain  Gain=Vnom/sqrt(3)*sqrt(2)  SaturateOnIntegerOverflow=on  OutDataTypeStr=Inherit: Same as input  ParamDataTypeStr=Inherit: Same as input
  to pu : Gain  Gain=(sqrt(2/3)*U_rated)
  "var->pu " : Gain  Gain=-1/Pnom  SaturateOnIntegerOverflow=on  OutDataTypeStr=Inherit: Same as input  ParamDataTypeStr=Inherit: Same as input
  Vdq_grid : Outport  VectorParamsAs1DForOutWhenUnconnected=off
  Idq_gc : Outport  Port=2  VectorParamsAs1DForOutWhenUnconnected=off
  "IL " : Outport  Port=3  VectorParamsAs1DForOutWhenUnconnected=off
  Flux : Outport  Port=4  VectorParamsAs1DForOutWhenUnconnected=off
  Vdc_meas : Outport  Port=5  VectorParamsAs1DForOutWhenUnconnected=off
  Pmeas : Outport  Port=6  VectorParamsAs1DForOutWhenUnconnected=off
  Qmeas : Outport  Port=7  VectorParamsAs1DForOutWhenUnconnected=off
  Vmeas : Outport  Port=8  VectorParamsAs1DForOutWhenUnconnected=off
  Theta_PLL : Outport  Port=9  VectorParamsAs1DForOutWhenUnconnected=off
  w_pu : Outport  Port=10  VectorParamsAs1DForOutWhenUnconnected=off
  "wr " : Outport  Port=11  VectorParamsAs1DForOutWhenUnconnected=off
  "Qref " : Outport  Port=12  VectorParamsAs1DForOutWhenUnconnected=off
  u_frt : Outport  Port=13
  u_f_protect : Outport  Port=14
  wires:
  Filter/9("angle_rotor ") -> [angle_rotor]
  angle_rotor/1 -> Filter/9(angle_rotor)
  Stator flux estimator/1(Flux) -> [Flux]
  # pairs of poles/1 -> Math Function/1
  Constant4/1 -> Math Function/2
  abc2qd/1(Vdq) -> [Vdqs]
  Trigonometric Function5/1 -> Mux2/2
  Trigonometric Function4/1 -> Mux2/1
  [angle_rotor] -> # pairs of poles/1
  [Vabc_LL_s] -> abc2qd/1(Vabc_LL)
  [sin_cos_rotor] -> abc2qd/2(sin_cos)
  Mux2/1 -> [sin_cos_rotor]
  Demux2/1 -> [Idqs]
  Demux2/2 -> Terminator2/1
  abc to dq2/1 -> Demux2/1
  [Iabc_s] -> abc to dq2/1
  [Vdqs] -> Stator flux estimator/1(Vdqs)
  [Idqs] -> Stator flux estimator/2(Idqs)
  [wr] -> Stator flux estimator/3(wr)
  [Qmeas] -> Qmeas/1
  "var->pu "/1 -> [Qmeas]
  [PQ] -> Selector3/1
  V->pu/1 -> [Vmeas]
  [V_volt] -> V->pu/1
  Selector2/1 -> [V_volt]
  Discrete 3-phase PLL-Driven Positive-Sequence Active & Reactive Power/1(Mag_V_I) -> Selector2/1
  Demux1/2 -> Terminator1/1
  Demux3/1 -> [Vdq_grid]
  Demux3/2 -> Terminator3/1
  abc to dq1/1 -> Demux1/1
  abc to dq0/1 -> Demux3/1
  PLL (3ph)/1 -> [Freq]
  Fnom/1 -> Divide3/2
  Divide3/1 -> [w_pu]
  pu->V/1 -> Scope/1, Discrete 3-phase PLL-Driven Positive-Sequence Active & Reactive Power/3(Vabc)
  W->pu/1 -> Scope/4, [Pmeas]
  [Freq] -> Divide3/1
  [Freq] -> Discrete 3-phase PLL-Driven Positive-Sequence Active & Reactive Power/1(Freq)
  PLL (3ph)/2 -> [Theta]
  [Vabc_grid] -> abc to dq0/1
  [Theta] -> Discrete 3-phase PLL-Driven Positive-Sequence Active & Reactive Power/2(w)
  [Theta] -> abc to dq0/2
  [Theta] -> abc to dq1/2
  [Vabc_grid] -> PLL (3ph)/1
  [Iabc_gc] -> abc to dq1/1
  [Theta] -> Theta_PLL/1
  Demux1/1 -> [Idq_gc]
  [Vdq_grid] -> Vdq_grid/1
  [Idq_gc] -> Idq_gc/1
  [w_pu] -> w_pu/1
  [Pmeas] -> Pmeas/1
  [Vmeas] -> Vmeas/1
  pu->A/1 -> Discrete 3-phase PLL-Driven Positive-Sequence Active & Reactive Power/4(Iabc), Scope/2
  [PQ] -> Selector1/1
  [Vdc_meas] -> Vdc_meas/1
  [Qref] -> "Qref "/1
  [wr] -> "wr "/1
  [Flux] -> Flux/1
  [Vabc_grid] -> pu->V/1
  [Iabc_gc] -> pu->A/1
  Discrete 3-phase PLL-Driven Positive-Sequence Active & Reactive Power/2(P_Q) -> Scope/3, [PQ]
  Vabc_grid/1 -> Filter/1(Vabc_grid)
  Vdc/1 -> Filter/6(Vdc)
  Qref/1 -> Filter/7(Qref)
  wr/1 -> Filter/8(wr)
  Filter/1("Vabc_grid ") -> [Vabc_grid]
  Filter/2("Iabc_grid_conv ") -> [Iabc_gc]
  Filter/4("Iabc_stator ") -> [Iabc_s]
  Filter/6("Vdc ") -> [Vdc_meas]
  Filter/8("wr ") -> [wr]
  Filter/7("Qref ") -> [Qref]
  Iabc_gc/1 -> Filter/2(Iabc_grid_conv)
  Iabc_s/1 -> Filter/4(Iabc_stator)
  Vabc_LL_s/1 -> Filter/3(Vabc_LL_s)
  Filter/3("Vabc_LL_s ") -> [Vabc_LL_s]
  [V_volt] -> Divide/1
  Constant1/1 -> Divide/2
  Divide/1 -> Math Function1/1
  Selector3/1 -> Sum/2
  C_var_filter/1 -> Sum/1
  Sum/1 -> "var->pu "/1
  Math Function1/1 -> C_var_filter/Q/1, C_var_filter/1
  Selector1/1 -> Sum1/1
  C_var_filter/Q/1 -> Sum1/2
  Sum1/1 -> W->pu/1
  IL/1 -> Filter/5(IL)
  Filter/5("IL ") -> [IL]
  [IL] -> "IL "/1
  Math Function/1 -> abc to dq2/2, Trigonometric Function5/1, Trigonometric Function4/1
  Extract References/1(u_frt_pu) -> [u_frt]
  Extract References/2(protection_u_f) -> [u_f_protect]
  [Vabc_grid] -> to pu/1
  [u_frt] -> u_frt/1
  [u_f_protect] -> u_f_protect/1
  to pu/1 -> Extract References/1(v_abc)

== system Auto_microgrid_forecasting_020322/Wind Turbine Type 4/Control/Speed & Pitch Control3 ==
  note: Current Regulator
  note: Note :
      | This control system is based on the report:
      | Dynamic Modeling of GE 1.5 and 3.6 Wind Turbine-Generators;
      | Prepared by: Nicholas W. Miller, William W. Price, Juan J. Sanchez-Gasca;
      | October 27, 2003, Version 3.0
      | GE-Power Systems Energy Consulting
      | Copyright 2002 General Electric Company, U.S.A.
      |
      | Another reference is:
      |
      | DYNAMIC MODELING OF GE 1.5 AND 3.6 MW WIND TURBINE GENERATORS
      | FOR STABILITY SIMULATIONS
      | Nicholas W. Miller, Juan J. Sanchez-Gasca, William W. Price Robert W. Delmerico
      | GE Power Systems GE Research
      | Schenectady, NY Niskayuna, NY
      |
      | 0-7803-7989-6/03/$17.00 02003 IEEE
  note: Speed Regulator
  note: Pitch Compensation
  note: Pitch Control
  wr : Inport
  Pmeas : Inport  Port=2
  IL : Inport  Port=3
  Tgain : Inport  Port=4
  Pref : Inport  Port=5
  U5s1 : Inport  Port=6
  0-inf : Saturate  UpperLimit=inf  LowerLimit=0
  0-pitch_max : Saturate  UpperLimit=pitch_max  LowerLimit=0
  "0-pitch_max " : Saturate  UpperLimit=pitch_max  LowerLimit=0
  Constant1 : Constant
  Delay1 : Delay  DelayLength=1  InitialCondition=2
  Discrete PI Controller1 : Subsystem  DialogController=POWERSYS.PowerSysDialog  mask(Discrete PI Controller){Kp=Kp_compensation, Ki=Ki_compensation, Par_Limits=[pitch_max 0], Init=0, Ts=Ts}
      mask prompts: Kp "Proportional gain (Kp):"; Ki "Integral gain (Ki):"; Par_Limits "Output limits: [ Upper   Lower ]"; Init "Output initial value:"; Ts "Sample time:"
      mask help: This block implements a discrete PI controller.
      mask init:
      | UpperLimit=Par_Limits(1);
      | LowerLimit=Par_Limits(2);
      | power_initmask();
      mask Help: This block is part of a subset of blocks in the Extras library that does not have documentation associated with it, other than the block mask description.
      mask Display: disp('PI');
  Discrete PI Controller2 : Subsystem  DialogController=POWERSYS.PowerSysDialog  mask(Discrete PI Controller){Kp=Kp_boost_cur_reg*1, Ki=Ki_boost_cur_reg*0.005, Par_Limits=[1 0], Init=0.5, Ts=Ts}
      mask prompts: Kp "Proportional gain (Kp):"; Ki "Integral gain (Ki):"; Par_Limits "Output limits: [ Upper   Lower ]"; Init "Output initial value:"; Ts "Sample time:"
      mask help: This block implements a discrete PI controller.
      mask init:
      | UpperLimit=Par_Limits(1);
      | LowerLimit=Par_Limits(2);
      | power_initmask();
      mask Help: This block is part of a subset of blocks in the Extras library that does not have documentation associated with it, other than the block mask description.
      mask Display: disp('PI');
  First-Order Filter : powerlib_meascontrol/Filters/First-Order Filter  FilterType=Lowpass  Tc=Pitch_time_constant  Ts=Ts  Initialize=on  Vac_Init=[0.8 -25 60]*0  Vdc_Init=0  PlotResponse=off  FreqRange="[0,  200,  1]"
      settings: SourceProductBaseCode=MT,PS
  First-Order Filter1 : powerlib_meascontrol/Filters/First-Order Filter  FilterType=Lowpass  Tc=T_speed  Ts=Ts  Initialize=on  Vac_Init=[0, 0, 0]  Vdc_Init=1+init(1)/100  PlotResponse=off  FreqRange="[0,  200,  1]"
      settings: SourceProductBaseCode=MT,PS
  Gain2 : Gain  Gain=Kp_pitch  SaturateOnIntegerOverflow=on  OutDataTypeStr=Inherit: Same as input  ParamDataTypeStr=Inherit: Same as input
  Less Than : RelationalOperator  Operator=<=  OutDataTypeStr=boolean  RndMeth=Simplest
  MATLAB Function1 : MATLAB Function  TreatAsAtomicUnit=on
  Merge1 : Merge  Inputs=3
  Operational1 : Subsystem  TreatAsAtomicUnit=on
  PID Controller1 : simulink/Continuous/PID Controller  Controller=PI  Form=Parallel  TimeDomain=Discrete-time  UseExternalTs=off  SampleTime=-1  IntegratorMethod=Forward Euler  FilterMethod=Forward Euler  ControllerParametersSource=internal  P=Kp_speed  I=Ki_speed  D=0  UseFilter=on  N=100  TunerSelectOption=Transfer Function Based (PID Tuner App)  InitialConditionSource=internal  InitialConditionForIntegrator=0  InitialConditionForFilter=0  DifferentiatorICPrevScaledInput=0  ExternalReset=none  TrackingMode=off  Kt=1  LimitOutput=on  UpperSaturationLimit=1.  LowerSaturationLimit=0.8  LinearizeAsGain=on  AntiWindupMode=back-calculation  Kb=1e4  POutMin=[]  POutMax=[]  IOutMin=[]  IOutMax=[]  DOutMin=[]  DOutMax=[]  NOutMin=[]  NOutMax=[]  SumOutMin=[]  SumOutMax=[]  SaturationOutMin=[]  SaturationOutMax=[]  PParamMin=[]  PParamMax=[]  IParamMin=[]  IParamMax=[]  DParamMin=[]  DParamMax=[]  NParamMin=[]  NParamMax=[]  KbParamMin=[]  KbParamMax=[]  KtParamMin=[]  KtParamMax=[]  KbOutMin=[]  KbOutMax=[]  KtOutMin=[]  KtOutMax=[]  IntegratorOutMin=[]  IntegratorOutMax=[]  FilterOutMin=[]  FilterOutMax=[]  SumI1OutMin=[]  SumI1OutMax=[]  SumI2OutMin=[]  SumI2OutMax=[]  SumI3OutMin=[]  SumI3OutMax=[]  SumI4OutMin=[]  SumI4OutMax=[]  SumDOutMin=[]  SumDOutMax=[]  DifferentiatorOutMin=[]  DifferentiatorOutMax=[]  FilterDiffOutCoefMin=[]  FilterDiffOutCoefMax=[]  ReciprocalOutMin=[]  ReciprocalOutMax=[]  SumDenOutMin=[]  SumDenOutMax=[]  SumNumOutMin=[]  SumNumOutMax=[]  DivideOutMin=[]  DivideOutMax=[]  UdiffTsProdOutMin=[]  UdiffTsProdOutMax=[]  NTsProdOutMin=[]  NTsProdOutMax=[]  UintegralTsProdOutMin=[]  UintegralTsProdOutMax=[]  UngainTsProdOutMin=[]  UngainTsProdOutMax=[]  IntegratorContinuousStateAttributes=''  IntegratorStateMustResolveToSignalObject=off  IntegratorRTWStateStorageClass=Auto  FilterContinuousStateAttributes=''  FilterStateMustResolveToSignalObject=off  FilterRTWStateStorageClass=Auto  ParallelPVariant=InternalParameters  IdealPVariant=Disabled  IVariant=InternalParameters  DVariant=Disabled  IntegratorVariant=Discrete  SatVariant=Enabled  AWVariant=BackCalculation  PCopyVariant=Disabled  TRVariant=Disabled  FdbkBlocksVariant=Forward  IdealPFdbkVariant=Disabled  SatFdbkVariant=Disabled  DerivativeFilterVariant=Disabled  NVariant=Disabled  NCopyVariant=Disabled_SignalSpec  FilterICVariant=Disabled  IntegratorICVariant=InternalICs  ExternalResetVariant=Disabled  TRSumVariant=Passthrough  SumFdbkVariant=Disabled  SumVariant=Sum_PI  TsampFilterVariant=InternalTs  TsampNgainVariant=Passthrough  TsampIntegralVariant=Passthrough
  Rate Limiter   1 : RateLimiter  RisingSlewLimit=pitch_rate  FallingSlewLimit=-pitch_rate
  Scope1 : Scope  NumInputPorts=6
  Scope4 : Scope  NumInputPorts=4
  Shutdown1 : Subsystem  TreatAsAtomicUnit=on
  Startup1 : Subsystem  TreatAsAtomicUnit=on
  Sum : Sum  Inputs=-+  SaturateOnIntegerOverflow=on
  Sum1 : Sum  Inputs=|+-
  Sum2 : Sum  Inputs=|+-  SaturateOnIntegerOverflow=on
  Sum3 : Sum  Inputs=|++
  Sum4 : Sum  Inputs=|+-
  Switch : Switch  Threshold=0.75
  Switch Case1 : SwitchCase  CaseConditions={1, 2, 3}
  Switch1 : Switch  Criteria=u2 > Threshold  Threshold=0.5
  Tracking Curve : Fcn  Expr=-0.5551*u(1)^2+1.183*u(1)+0.425
  pu_elec->pu_mec : Gain  Gain=Pnom/Pmec
  wref : Constant
  Duty_Cycle : Outport  VectorParamsAs1DForOutWhenUnconnected=off
  Pitch (deg) : Outport  Port=2  VectorParamsAs1DForOutWhenUnconnected=off
  wires:
  First-Order Filter/1 -> Operational1/1(In1)  "Pitch"
  MATLAB Function1/1(state) -> Delay1/1, Scope4/1, Switch Case1/1  "state"
  Delay1/1 -> MATLAB Function1/3("state ")
  Switch Case1/1 -> Startup1/Action
  Startup1/1(Out1) -> Merge1/1
  [wr] -> MATLAB Function1/2(wr), Scope4/3  "wr"
  U5s1/1 -> MATLAB Function1/1(U5s), Scope4/2  "U5s"
  Switch Case1/2 -> Operational1/Action
  Merge1/1 -> Pitch (deg)/1, Scope4/4  "pitch"
  Shutdown1/1(Out1) -> Merge1/3
  Switch Case1/3 -> Shutdown1/Action
  Operational1/1(Out1) -> Merge1/2
  PID Controller1/1 -> Switch1/1  "ILref"
  Less Than/1 -> Switch1/2
  Constant1/1 -> Less Than/2
  Tgain/1 -> Less Than/1, Switch1/3
  Switch1/1 -> Sum4/1, Scope1/4  "ILref"
  Discrete PI Controller2/1(Out) -> Duty_Cycle/1, Scope1/6  "Duty cycle"
  IL/1 -> Sum4/2, Scope1/5  "IL"
  Sum4/1 -> Discrete PI Controller2/1(Error)
  Tracking Curve/1 -> Switch/3
  First-Order Filter1/1 -> Sum/1, Sum1/2, Scope1/1  "wref"
  Sum2/1 -> Discrete PI Controller1/1(Error)
  Sum/1 -> Gain2/1
  "0-pitch_max "/1 -> First-Order Filter/1
  0-pitch_max/1 -> Sum3/1  "Pitch_contrl"
  Pmeas/1 -> 0-inf/1
  Discrete PI Controller1/1(Out) -> Sum3/2  "Pitch_comp"
  Gain2/1 -> 0-pitch_max/1
  Rate Limiter   1/1 -> "0-pitch_max "/1
  Sum3/1 -> Rate Limiter   1/1
  Pref/1 -> Sum2/2  "Pref"
  Sum1/1 -> Scope1/3, PID Controller1/1  "wdiff"
  Switch/1 -> First-Order Filter1/1
  wref/1 -> Switch/1
  pu_elec->pu_mec/1 -> Switch/2, Sum2/1, Tracking Curve/1  "Pmes"
  0-inf/1 -> pu_elec->pu_mec/1
  wr/1 -> Sum1/1, Sum/2, [wr], Scope1/2  "wr"
